simulink model "parameter_sweep_LR"  (R2020a)
settings: Solver=VariableStepAuto  StartTime=0.0  StopTime=10.0  RelTol=1e-3
values from neighbouring files (symbols this model uses):
  R = 4.95    [parameter_sweep_LRM_plotter.m]    (also in parameter_sweep_LR_plotter.m = 7; parameter_sweep_M_plotter.m = 7; parameter_sweep_Mechanical_plotter.m = 5)
  R_Int = 0.55    [parameter_sweep_LRM_plotter.m]    (also in parameter_sweep_Mechanical_plotter.m = 0.33)
  V_T = 33.5    [parameter_sweep_LRM_plotter.m]    (also in parameter_sweep_LR_plotter.m = 4 + ((i-1) * 1); parameter_sweep_M_plotter.m = 350; parameter_sweep_Mechanical_plotter.m)
libraries: fl_lib x8, nesl_utility x7
settings Model: Creator=insat  LastModifiedBy=gwb15193

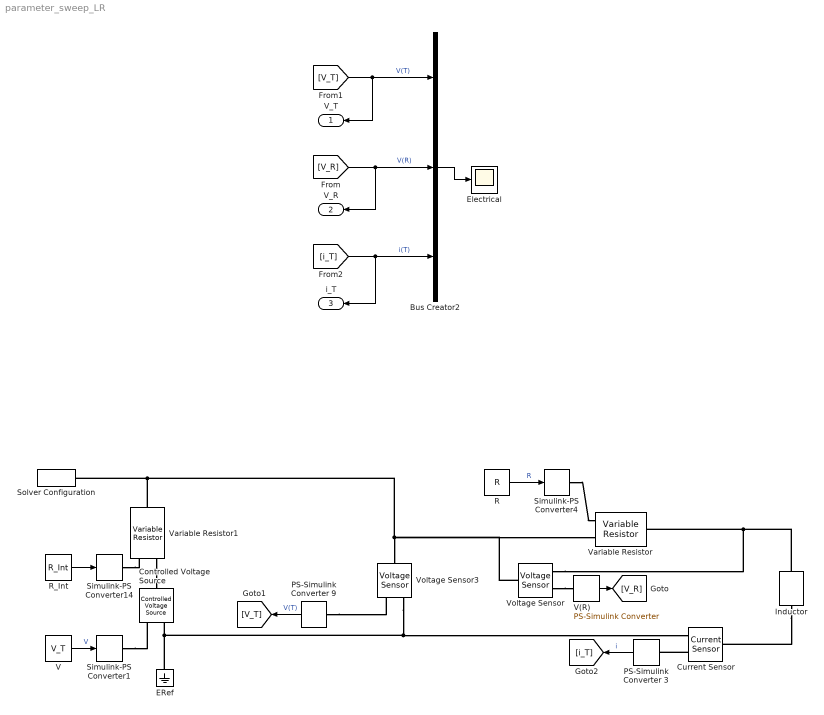
== system parameter_sweep_LR ==
  Bus Creator2 : BusCreator  Inputs=3
  Controlled Voltage Source : fl_lib/Electrical/Electrical Sources/Controlled Voltage Source
  Current Sensor : fl_lib/Electrical/Electrical Sensors/Current Sensor
  ERef : fl_lib/Electrical/Electrical Elements/Electrical Reference
  Electrical : Scope
  Inductor : fl_lib/Electrical/Electrical Elements/Inductor  l=1 H  r=0 Ohm  g=1e-16 1/Ohm  i_specify=off  i_priority=None  i=0 A  i_nominal_specify=off  i_nominal_unit=A  i_nominal_value=1  v_specify=off  v_priority=None  v=0 V  v_nominal_specify=off  v_nominal_unit=V  v_nominal_value=1  i_L_specify=off  i_L_priority=High  i_L=0 A  i_L_nominal_specify=off  i_L_nominal_unit=A  i_L_nominal_value=1
  PS-Simulink Converter 3 : nesl_utility/PS-Simulink Converter  PhysicalDomain=network_engine_domain  SubClassName=ps_output  LeftPortType=input  RightPortType=output  PseudoPeriodic=off  Frequencies=[]  Unit=A  AffineConversion=off
  PS-Simulink Converter 9 : nesl_utility/PS-Simulink Converter  PhysicalDomain=network_engine_domain  SubClassName=ps_output  LeftPortType=input  RightPortType=output  PseudoPeriodic=off  Frequencies=[]  Unit=V  AffineConversion=off
  R : Constant  Value=R
  R_Int : Constant  Value=R_Int
  Simulink-PS Converter1 : nesl_utility/Simulink-PS Converter  PhysicalDomain=network_engine_domain  SubClassName=ps_input  LeftPortType=input  RightPortType=output  PseudoPeriodic=off  Frequencies=[]  NoiseDistribution=none  NoiseParameters=[]  Unit=1  AffineConversion=off  FilteringAndDerivatives=zero  SimscapeFilterOrder=1  InputFilterTimeConstant=.001  UdotUserProvided=0
  Simulink-PS Converter14 : nesl_utility/Simulink-PS Converter  PhysicalDomain=network_engine_domain  SubClassName=ps_input  LeftPortType=input  RightPortType=output  PseudoPeriodic=off  Frequencies=[]  NoiseDistribution=none  NoiseParameters=[]  Unit=1  AffineConversion=off  FilteringAndDerivatives=zero  SimscapeFilterOrder=1  InputFilterTimeConstant=.001  UdotUserProvided=0
  Simulink-PS Converter4 : nesl_utility/Simulink-PS Converter  PhysicalDomain=network_engine_domain  SubClassName=ps_input  LeftPortType=input  RightPortType=output  PseudoPeriodic=off  Frequencies=[]  NoiseDistribution=none  NoiseParameters=[]  Unit=1  AffineConversion=off  FilteringAndDerivatives=zero  SimscapeFilterOrder=1  InputFilterTimeConstant=.001  UdotUserProvided=0
  Solver Configuration : nesl_utility/Solver Configuration  PhysicalDomain=network_engine_domain  SubClassName=solver  LeftPortType=input  RightPortType=generic  Tones=[]  Harmonics=[]  SimulateNoise=off  Profile=off  UseLocalSampling=off  EnableSwitchedLinearOptims=on  FrequencyDomain=off  UseCCode=off  RelTol=0.001  AbsTol=1e-06  MinStep=1e-09  ToWorkspace=off  RevertToSquareIcSolve=off  NumHomotopyIterations=100  PhasorMode=off  PhasorModeNumHarmonics=1  DoDC=off  ResidualTolerance=1e-9  UseLocalSolver=off  LocalSolverChoice=NE_BACKWARD_EULER_ADVANCER  LocalSolverSampleTime=.001  DoFixedCost=off  MaxNonlinIter=3  MaxModeIter=2  LinearAlgebra=auto  EquationFormulation=NE_TIME_EF  DelaysMemoryBudget=1024  AutomaticFiltering=on  FilteringTimeConstant=0.0001  PartitionStorageMethod=AS_NEEDED  PartitionMemoryBudget=1024  PartitionMethod=FAST
  V : Constant  Value=V_T
  V(R) : nesl_utility/PS-Simulink Converter  PhysicalDomain=network_engine_domain  SubClassName=ps_output  LeftPortType=input  RightPortType=output  PseudoPeriodic=off  Frequencies=[]  Unit=V  AffineConversion=off
  Variable Resistor : fl_lib/Electrical/Electrical Elements/Variable Resistor  Rmin=0 Ohm  i_specify=off  i_priority=None  i=0 A  i_nominal_specify=off  i_nominal_unit=A  i_nominal_value=1  v_specify=off  v_priority=None  v=0 V  v_nominal_specify=off  v_nominal_unit=V  v_nominal_value=1
  Variable Resistor1 : fl_lib/Electrical/Electrical Elements/Variable Resistor  Rmin=0 Ohm  i_specify=off  i_priority=None  i=0 A  i_nominal_specify=off  i_nominal_unit=A  i_nominal_value=1  v_specify=off  v_priority=None  v=0 V  v_nominal_specify=off  v_nominal_unit=V  v_nominal_value=1
  Voltage Sensor : fl_lib/Electrical/Electrical Sensors/Voltage Sensor
  Voltage Sensor3 : fl_lib/Electrical/Electrical Sensors/Voltage Sensor
  V_T : Outport  SignalName=V_T
  V_R : Outport  Port=2  SignalName=V_R
  i_T : Outport  Port=3  SignalName=i_T
  wires:
  V(R)/1 -> [V_R]
  R/1 -> Simulink-PS Converter4/1  "R"
  PS-Simulink Converter 3/1 -> [i_T]  "i"
  PS-Simulink Converter 9/1 -> [V_T]  "V(T)"
  Bus Creator2/1 -> Electrical/1
  [i_T] -> i_T/1, Bus Creator2/3  "i(T)"
  [V_T] -> V_T/1, Bus Creator2/1  "V(T)"
  [V_R] -> V_R/1, Bus Creator2/2  "V(R)"
  V/1 -> Simulink-PS Converter1/1  "V"
  R_Int/1 -> Simulink-PS Converter14/1
  connections:
  Voltage Sensor/RConn2 -- Inductor/RConn1 -- Variable Resistor/RConn1
  Current Sensor/RConn1 -- PS-Simulink Converter 3/LConn1
  Voltage Sensor/RConn1 -- V(R)/LConn1
  PS-Simulink Converter 9/LConn1 -- Voltage Sensor3/RConn1
  Simulink-PS Converter4/RConn1 -- Variable Resistor/LConn1
  Inductor/LConn1 -- Current Sensor/LConn1
  Voltage Sensor3/RConn2 -- ERef/LConn1 -- Controlled Voltage Source/RConn2 -- Current Sensor/RConn2
  Voltage Sensor/LConn1 -- Variable Resistor/LConn2 -- Variable Resistor1/RConn1 -- Solver Configuration/RConn1 -- Voltage Sensor3/LConn1
  Variable Resistor1/LConn2 -- Controlled Voltage Source/LConn1
  Simulink-PS Converter1/RConn1 -- Controlled Voltage Source/RConn1
  Simulink-PS Converter14/RConn1 -- Variable Resistor1/LConn1
